simulink model "full_order_rearranged_to_pdf"  (R2015b)
settings: Solver=VariableStepAuto  StartTime=0.0  StopTime=10.0  RelTol=1e-3
undefined symbols (not defined in the file): c_drag_pro, Iq, J_pro, Kt, L, R
libraries: simulink x1
settings Model: Creator=Morten  LastModifiedBy=Morten

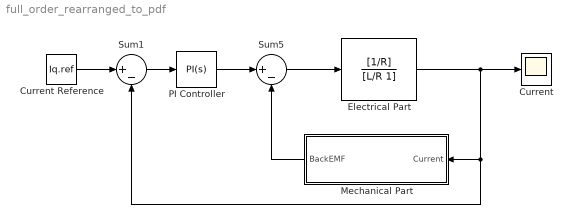
== system full_order_rearranged_to_pdf ==
  Current Reference : Constant  Value=Iq.ref
  "Current " : Scope
  Electrical Part : TransferFcn  Numerator=[1/R]  Denominator=[L/R 1]
  "Mechanical Part " : Subsystem
  PI Controller : simulink/Continuous/PID Controller  Controller=PI  TimeDomain=Continuous-time  SampleTime=-1  IntegratorMethod=Forward Euler  FilterMethod=Forward Euler  Form=Parallel  UseFilter=on  ControllerParametersSource=internal  P=0.0039  I=0.4606  D=0  N=100  InitialConditionSource=internal  InitialConditionForIntegrator=0  InitialConditionForFilter=0  ExternalReset=none  LimitOutput=off  UpperSaturationLimit=inf  LowerSaturationLimit=-inf  LinearizeAsGain=on  AntiWindupMode=none  Kb=1  TrackingMode=off  Kt=1  PParamMin=[]  PParamMax=[]  IParamMin=[]  IParamMax=[]  DParamMin=[]  DParamMax=[]  NParamMin=[]  NParamMax=[]  KbParamMin=[]  KbParamMax=[]  KtParamMin=[]  KtParamMax=[]  POutMin=[]  POutMax=[]  IOutMin=[]  IOutMax=[]  DOutMin=[]  DOutMax=[]  NOutMin=[]  NOutMax=[]  KbOutMin=[]  KbOutMax=[]  KtOutMin=[]  KtOutMax=[]  IntegratorOutMin=[]  IntegratorOutMax=[]  FilterOutMin=[]  FilterOutMax=[]  SumOutMin=[]  SumOutMax=[]  SumI1OutMin=[]  SumI1OutMax=[]  SumI2OutMin=[]  SumI2OutMax=[]  SumI3OutMin=[]  SumI3OutMax=[]  SumDOutMin=[]  SumDOutMax=[]  SaturationOutMin=[]  SaturationOutMax=[]  IntegratorContinuousStateAttributes=''  IntegratorStateMustResolveToSignalObject=off  IntegratorRTWStateStorageClass=Auto  FilterContinuousStateAttributes=''  FilterStateMustResolveToSignalObject=off  FilterRTWStateStorageClass=Auto  DifferentiatorICPrevScaledInput=0  DifferentiatorOutMin=[]  DifferentiatorOutMax=[]
  Sum1 : Sum  Inputs=|+-
  Sum5 : Sum  Inputs=|+-
  wires:
  PI Controller/1 -> Sum5/1
  Sum1/1 -> PI Controller/1
  Current Reference/1 -> Sum1/1
  "Mechanical Part "/1(BackEMF) -> Sum5/2
  Sum5/1 -> Electrical Part/1
  Electrical Part/1 -> Sum1/2, "Mechanical Part "/1(Current), "Current "/1

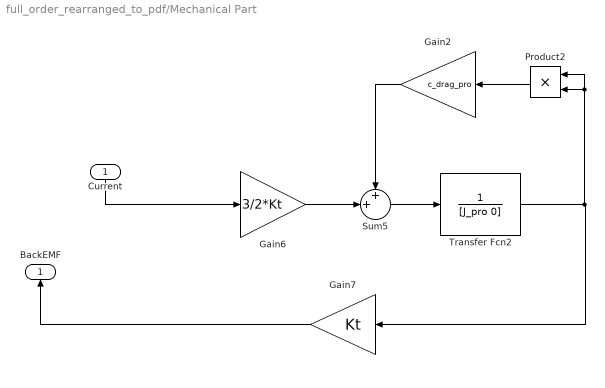
== system full_order_rearranged_to_pdf/Mechanical Part  ==
  Current : Inport
  Gain2 : Gain  Gain=c_drag_pro
  Gain6 : Gain  Gain=3/2*Kt
  Gain7 : Gain  Gain=Kt
  Product2 : Product
  Sum5 : Sum  Inputs=++|
  Transfer Fcn2 : TransferFcn  Denominator=[J_pro 0]
  BackEMF : Outport
  wires:
  Gain6/1 -> Sum5/2
  Transfer Fcn2/1 -> Product2/2, Product2/1, Gain7/1
  Gain2/1 -> Sum5/1
  Sum5/1 -> Transfer Fcn2/1
  Product2/1 -> Gain2/1
  Gain7/1 -> BackEMF/1
  Current/1 -> Gain6/1
